simulink model "Riego"  (R2020a)
settings: Solver=VariableStepAuto  StartTime=0.0  StopTime=10.0  RelTol=1e-3
settings Model: Creator=sergi  LastModifiedBy=sergi

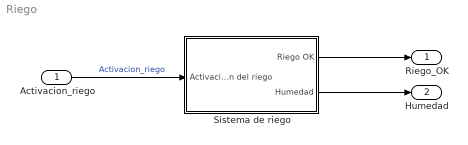
== system Riego ==
  Activacion_riego : Inport  PortDimensions=1
  Sistema de riego : Subsystem
  Riego_OK : Outport  VectorParamsAs1DForOutWhenUnconnected=off
  Humedad : Outport  Port=2  VectorParamsAs1DForOutWhenUnconnected=off
  wires:
  Activacion_riego/1 -> Sistema de riego/1(Activacion del riego)  "Activacion_riego"
  Sistema de riego/1(Riego OK) -> Riego_OK/1
  Sistema de riego/2(Humedad) -> Humedad/1

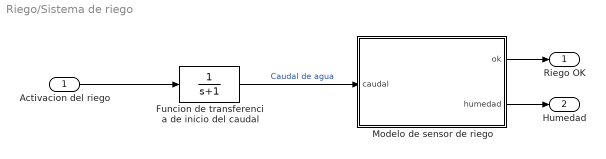
== system Riego/Sistema de riego ==
  Activacion del riego : Inport
  Funcion de transferencia de inicio del caudal : TransferFcn  Denominator=[1 1]
  Modelo de sensor de riego : MATLAB Function  TreatAsAtomicUnit=on
  Riego OK : Outport
  Humedad : Outport  Port=2
  wires:
  Activacion del riego/1 -> Funcion de transferencia de inicio del caudal/1
  Funcion de transferencia de inicio del caudal/1 -> Modelo de sensor de riego/1(caudal)  "Caudal de agua"
  Modelo de sensor de riego/1(ok) -> Riego OK/1
  Modelo de sensor de riego/2(humedad) -> Humedad/1

== matlab function Riego/Sistema de riego/Modelo de sensor de riego ==
  data: caudal input; ok output; humedad output
function [ok, humedad] = Modelo_Riego(caudal)
persistent humedad_
if isempty(agua)
    agua = 0;
    humedad_ = 0;
end

agua = agua + caudal;

humedad = agua/100;

if humedad > 1
    humedad = 1;
end

if humedad_ < humedad
    ok = 1;
else
    ok = 0;
end
